simulink model "simple_model"  (R2019a)
settings: Solver=VariableStepAuto  StartTime=0.0  StopTime=10.0  RelTol=1e-3
settings Model: Creator=amah2  LastModifiedBy=amah2

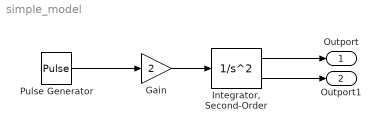
== system simple_model ==
  Gain : Gain  Gain=2
  "Integrator, Second-Order" : SecondOrderIntegrator  ICX=0
  Pulse Generator : DiscretePulseGenerator  PulseType=Time based  Period=10  PulseWidth=5
  Outport : Outport
  Outport1 : Outport  Port=2
  wires:
  Pulse Generator/1 -> Gain/1
  Gain/1 -> "Integrator, Second-Order"/1
  "Integrator, Second-Order"/1 -> Outport/1
  "Integrator, Second-Order"/2 -> Outport1/1
